simulink model "WaveletTraj"  (Simulink 10.1)
settings: Solver=FixedStepDiscrete  StartTime=0.0  StopTime=inf  FixedStep=Ts  RelTol=1e-3
PreLoadFcn:
  | load param
undefined symbols (not defined in the file or in its folder): c_maxsz, DiscIntNeverNeededParam, Dphival_fi, f, interp_gain, interp_uplim, phival_fi, Ts, tval_fi, w
libraries: simulink x36, dspsigops x24, dspindex x16, dspswit3 x12, simulink_extras x8
(part 3 of 4)

== system WaveletTraj/Wavelet Trajectory/TrajGen1/Compute Join Output/CalcRho ==
  tau : Inport
  tau1 : Inport  Port=2
  Constant : Constant  OutDataTypeStr=fixdt(1,w,f)
  Divide : Product  Inputs=*/  OutDataTypeStr=fixdt(1,w,f)  RndMeth=Nearest  SaturateOnIntegerOverflow=on
  Product : Product  OutDataTypeStr=fixdt(1,w,f)  RndMeth=Nearest  SaturateOnIntegerOverflow=on
  Saturation1 : Saturate  UpperLimit=2^(w-f-1)  LowerLimit=2^-f  OutDataTypeStr=fixdt(1,w,f)  RndMeth=Nearest
  Sum1 : Sum  Inputs=|+-  OutDataTypeStr=fixdt(1,w,f)  RndMeth=Nearest  SaturateOnIntegerOverflow=on
  Sum2 : Sum  Inputs=-+|  OutDataTypeStr=fixdt(1,w,f)  RndMeth=Nearest  SaturateOnIntegerOverflow=on
  Rho1 : Outport
  Rho2 : Outport  Port=2
  wires:
  Sum2/1 -> Rho2/1
  Saturation1/1 -> Divide/2
  Product/1 -> Sum2/1, Rho1/1
  Sum1/1 -> Product/2, Product/1
  Constant/1 -> Sum2/2, Sum1/2
  Divide/1 -> Sum1/1
  tau1/1 -> Saturation1/1
  tau/1 -> Divide/1

== system WaveletTraj/Wavelet Trajectory/TrajGen1/Compute Outputs/Compute Integral ==
  x : Inport
  max : Inport  Port=2
  min : Inport  Port=3
  Enable : EnablePort
  Compare To Zero : simulink/Logic and Bit Operations/Compare To Zero  SystemSampleTime=-1  relop=<  LogicOutDataTypeMode=boolean  ZeroCross=off
  Compare To Zero1 : simulink/Logic and Bit Operations/Compare To Zero  SystemSampleTime=-1  relop=>  LogicOutDataTypeMode=boolean  ZeroCross=off
  Discrete-Time Integrator : DiscreteIntegrator  IntegratorMethod=Integration: Trapezoidal  ExternalReset=level  InitialConditionSource=external  SampleTime=Ts  OutDataTypeStr=fixdt(1,w,f)  RndMeth=Nearest  SaturateOnIntegerOverflow=on  ICPrevOutput=DiscIntNeverNeededParam  ICPrevScaledInput=DiscIntNeverNeededParam
  Logical Operator : Logic  Operator=OR  IconShape=distinctive  AllPortsSameDT=off  OutDataTypeStr=boolean
  Logical Operator1 : Logic  IconShape=distinctive  AllPortsSameDT=off  OutDataTypeStr=boolean
  Logical Operator2 : Logic  IconShape=distinctive  AllPortsSameDT=off  OutDataTypeStr=boolean
  Logical Operator3 : Logic  Operator=OR  IconShape=distinctive  AllPortsSameDT=off  OutDataTypeStr=boolean
  Relational Operator1 : RelationalOperator  Operator=<=  OutDataTypeStr=boolean  RndMeth=Nearest
  Relational Operator2 : RelationalOperator  Operator=<=  OutDataTypeStr=boolean  RndMeth=Nearest
  S-R Flip-Flop : simulink_extras/Flip Flops/S-R Flip-Flop  SystemSampleTime=-1  initial_condition=0
  Sample and Hold1 : dspsigops/Sample and Hold  SystemSampleTime=-1  trig=Either edge  initCond=0  latchinput=off
  Sample and Hold2 : dspsigops/Sample and Hold  SystemSampleTime=-1  trig=Either edge  initCond=0  latchinput=off
  Saturation Dynamic : simulink/Discontinuities/Saturation Dynamic  SystemSampleTime=-1  OutMin=[]  OutMax=[]  OutDataTypeStr=fixdt(1,w,f)  OutputDataTypeScalingMode=Specify via dialog  OutDataType=fixdt(1,w,f)  OutScaling=[]  RndMeth=Nearest  DoSatur=on
  Terminator : Terminator
  Unit Delay : UnitDelay  SampleTime=-1
  Ix : Outport
  wires:
  max/1 -> Relational Operator1/1, Saturation Dynamic/1
  min/1 -> Relational Operator2/2, Saturation Dynamic/3
  Relational Operator1/1 -> Logical Operator/1, Sample and Hold1/1
  Relational Operator2/1 -> Sample and Hold2/1, Logical Operator/2
  Discrete-Time Integrator/1 -> Saturation Dynamic/2
  Saturation Dynamic/1 -> Ix/1, Unit Delay/1
  x/1 -> Discrete-Time Integrator/1, Compare To Zero/1, Compare To Zero1/1
  Unit Delay/1 -> Discrete-Time Integrator/3, Relational Operator1/2, Relational Operator2/1
  S-R Flip-Flop/1 -> Discrete-Time Integrator/2
  S-R Flip-Flop/2 -> Terminator/1
  Logical Operator/1 -> S-R Flip-Flop/1, Sample and Hold1/Trigger, Sample and Hold2/Trigger
  Compare To Zero/1 -> Logical Operator1/2
  Compare To Zero1/1 -> Logical Operator2/2
  Logical Operator1/1 -> Logical Operator3/1
  Logical Operator2/1 -> Logical Operator3/2
  Logical Operator3/1 -> S-R Flip-Flop/2
  Sample and Hold1/1 -> Logical Operator1/1
  Sample and Hold2/1 -> Logical Operator2/1

== system WaveletTraj/Wavelet Trajectory/TrajGen1/Compute Outputs/Rate Limiter1 ==
  up : Inport
  u : Inport  Port=2
  lo : Inport  Port=3
  Gain : Gain  Gain=1/Ts  ParamDataTypeStr=fixdt(1,w,f)  RndMeth=Nearest  SaturateOnIntegerOverflow=on  OutDataTypeStr=Inherit: Same as input
  Gain1 : Gain  Gain=Ts  ParamDataTypeStr=fixdt(1,w,f)  OutDataTypeStr=fixdt(1,w,f)  RndMeth=Nearest  SaturateOnIntegerOverflow=on
  Gain2 : Gain  Gain=Ts  ParamDataTypeStr=fixdt(1,w,f)  OutDataTypeStr=fixdt(1,w,f)  RndMeth=Nearest  SaturateOnIntegerOverflow=on
  Relational Operator : RelationalOperator  Operator=<  OutDataTypeStr=boolean  RndMeth=Nearest
  Relational Operator1 : RelationalOperator  Operator=>  OutDataTypeStr=boolean  RndMeth=Nearest
  Sum1 : Sum  Inputs=|++  OutDataTypeStr=fixdt(1,w,f)  RndMeth=Nearest  SaturateOnIntegerOverflow=on
  Sum2 : Sum  Inputs=|+-  OutDataTypeStr=fixdt(1,w,f)  RndMeth=Nearest  SaturateOnIntegerOverflow=on
  Sum3 : Sum  Inputs=|++  OutDataTypeStr=fixdt(1,w,f)  RndMeth=Nearest  SaturateOnIntegerOverflow=on
  Switch1 : Switch  Threshold=0.5  OutDataTypeStr=fixdt(1,w,f)  RndMeth=Nearest  SaturateOnIntegerOverflow=on
  Switch2 : Switch  Threshold=0.5  OutDataTypeStr=fixdt(1,w,f)  RndMeth=Nearest  SaturateOnIntegerOverflow=on
  Unit Delay : UnitDelay  SampleTime=-1
  y : Outport
  wires:
  u/1 -> Sum2/1, Switch1/3
  Sum2/1 -> Gain/1
  Unit Delay/1 -> Sum2/2, Sum1/2, Sum3/2
  Gain/1 -> Relational Operator/2, Relational Operator1/1
  up/1 -> Relational Operator/1, Gain1/1
  Relational Operator/1 -> Switch1/2
  Gain1/1 -> Sum1/1
  Sum1/1 -> Switch1/1
  Switch1/1 -> Switch2/1
  Switch2/1 -> y/1, Unit Delay/1
  Relational Operator1/1 -> Switch2/2
  lo/1 -> Relational Operator1/2, Gain2/1
  Gain2/1 -> Sum3/1
  Sum3/1 -> Switch2/3

== system WaveletTraj/Wavelet Trajectory/TrajGen1/Compute Outputs/Rate Limiter2 ==
  up : Inport
  u : Inport  Port=2
  lo : Inport  Port=3
  Gain : Gain  Gain=1/Ts  ParamDataTypeStr=fixdt(1,w,f)  RndMeth=Nearest  SaturateOnIntegerOverflow=on  OutDataTypeStr=Inherit: Same as input
  Gain1 : Gain  Gain=Ts  ParamDataTypeStr=fixdt(1,w,f)  OutDataTypeStr=fixdt(1,w,f)  RndMeth=Nearest  SaturateOnIntegerOverflow=on
  Gain2 : Gain  Gain=Ts  ParamDataTypeStr=fixdt(1,w,f)  OutDataTypeStr=fixdt(1,w,f)  RndMeth=Nearest  SaturateOnIntegerOverflow=on
  Relational Operator : RelationalOperator  Operator=<  OutDataTypeStr=boolean  RndMeth=Nearest
  Relational Operator1 : RelationalOperator  Operator=>  OutDataTypeStr=boolean  RndMeth=Nearest
  Sum1 : Sum  Inputs=|++  OutDataTypeStr=fixdt(1,w,f)  RndMeth=Nearest  SaturateOnIntegerOverflow=on
  Sum2 : Sum  Inputs=|+-  OutDataTypeStr=fixdt(1,w,f)  RndMeth=Nearest  SaturateOnIntegerOverflow=on
  Sum3 : Sum  Inputs=|++  OutDataTypeStr=fixdt(1,w,f)  RndMeth=Nearest  SaturateOnIntegerOverflow=on
  Switch1 : Switch  Threshold=0.5  OutDataTypeStr=fixdt(1,w,f)  RndMeth=Nearest  SaturateOnIntegerOverflow=on
  Switch2 : Switch  Threshold=0.5  OutDataTypeStr=fixdt(1,w,f)  RndMeth=Nearest  SaturateOnIntegerOverflow=on
  Unit Delay : UnitDelay  SampleTime=-1
  y : Outport
  wires:
  Sum3/1 -> Switch2/3
  Gain2/1 -> Sum3/1
  lo/1 -> Gain2/1, Relational Operator1/2
  Relational Operator1/1 -> Switch2/2
  Switch2/1 -> Unit Delay/1, y/1
  Switch1/1 -> Switch2/1
  Sum1/1 -> Switch1/1
  Gain1/1 -> Sum1/1
  Relational Operator/1 -> Switch1/2
  up/1 -> Gain1/1, Relational Operator/1
  Gain/1 -> Relational Operator1/1, Relational Operator/2
  Unit Delay/1 -> Sum3/2, Sum1/2, Sum2/2
  Sum2/1 -> Gain/1
  u/1 -> Switch1/3, Sum2/1

== system WaveletTraj/Wavelet Trajectory/TrajGen1/Compute Position/Position ==
  Res : Inport
  tau : Inport  Port=2
  c : Inport  Port=3
  N : Inport  Port=4
  Position : Subsystem  RTWFcnName=Trajectory_Position
  out : Outport
  wires:
  N/1 -> Position/4(N)
  c/1 -> Position/3(c)
  Position/1(out) -> out/1
  tau/1 -> Position/2(tau)
  Res/1 -> Position/1(Res)

== system WaveletTraj/Wavelet Trajectory/TrajGen1/Input Latching/Sample and Hold ==
  mode : Inport
  In : Inport  Port=2
  Trigger : TriggerPort  VariantControl=(inherit)  ZeroCross=off
  Constant : Constant  Value=2^3  OutDataTypeStr=fixdt(0,w,f)
  Constant1 : Constant  Value=2^4  OutDataTypeStr=fixdt(0,w,f)
  Data Type Conversion : DataTypeConversion  OutDataTypeStr=uint16  RndMeth=Ceiling  SaturateOnIntegerOverflow=on
  Multiport Switch : MultiPortSwitch  DataPortOrder=Zero-based contiguous  zeroidx=on  OutDataTypeStr=fixdt(0,w,f)  RndMeth=Nearest  SaturateOnIntegerOverflow=on
  " " : Outport  InitialOutput=initCond
  " 1" : Outport  Port=2  InitialOutput=initCond
  wires:
  Data Type Conversion/1 -> " 1"/1
  Multiport Switch/1 -> " "/1, Data Type Conversion/1
  mode/1 -> Multiport Switch/1
  In/1 -> Multiport Switch/2
  Constant/1 -> Multiport Switch/3
  Constant1/1 -> Multiport Switch/4

== system WaveletTraj/Wavelet Trajectory/TrajGen1/Input Latching/Sample and Hold2 ==
  In : Inport
  Trigger : TriggerPort  VariantControl=(inherit)  ZeroCross=off
  Data Type Conversion : DataTypeConversion  OutDataTypeStr=uint32  SaturateOnIntegerOverflow=on
  Gain : Gain  Gain=1/Ts  ParamDataTypeStr=fixdt(1,w,f)  OutDataTypeStr=fixdt(1,w,f)  RndMeth=Nearest  SaturateOnIntegerOverflow=on
  " " : Outport  InitialOutput=initCond
  wires:
  Data Type Conversion/1 -> " "/1
  Gain/1 -> Data Type Conversion/1
  In/1 -> Gain/1

== system WaveletTraj/Wavelet Trajectory/TrajGen1/Input Latching/Sample and Hold4 ==
  mode : Inport
  In : Inport  Port=2
  Trigger : TriggerPort  VariantControl=(inherit)  ZeroCross=off
  Multiport Switch : MultiPortSwitch  DataPortOrder=Zero-based contiguous  zeroidx=on  OutDataTypeStr=fixdt(1,w,f)  RndMeth=Nearest  SaturateOnIntegerOverflow=on
  constant : Constant  Value="[0.0156906989743308,  0.104549075132343,  0.277142440037961,  0.502199121925297,  0.726584938978675,  0.897421193763573,  0.982811374526835,  0.999579465917557,  1.00001660256494,  zeros(1,c_maxsz-9)]"  OutDataTypeStr=fixdt(1,w,f)
  constant1 : Constant  Value="[0.704980465851185,  0.994792363880808,  1.00001660256494*ones(1,15),  zeros(1,c_maxsz-17)]"  OutDataTypeStr=fixdt(1,w,f)
  " " : Outport  InitialOutput=initCond
  wires:
  Multiport Switch/1 -> " "/1
  mode/1 -> Multiport Switch/1
  In/1 -> Multiport Switch/2
  constant/1 -> Multiport Switch/3
  constant1/1 -> Multiport Switch/4

== system WaveletTraj/Wavelet Trajectory/TrajGen1/Input Latching/Sample and Hold5 ==
  mode : Inport
  x0 : Inport  Port=2
  xf : Inport  Port=3
  Trigger : TriggerPort  VariantControl=(inherit)  ZeroCross=off
  Constant : Constant  OutDataTypeStr=fixdt(1,w,f)
  Sum2 : Sum  Inputs=-+|  OutDataTypeStr=fixdt(1,w,f)  RndMeth=Nearest  SaturateOnIntegerOverflow=on
  Switch1 : Switch  Threshold=0.5  OutDataTypeStr=fixdt(1,w,f)  RndMeth=Nearest  SaturateOnIntegerOverflow=on
  " " : Outport  InitialOutput=initCond
  wires:
  x0/1 -> Sum2/1
  xf/1 -> Sum2/2
  mode/1 -> Switch1/2
  Sum2/1 -> Switch1/1
  Switch1/1 -> " "/1
  Constant/1 -> Switch1/3

== system WaveletTraj/Wavelet Trajectory/TrajGen2/Compute Join Coeffs/Derivative1 in tau ==
  Res : Inport
  tau : Inport  Port=2
  c : Inport  Port=3
  N : Inport  Port=4
  Derivative : Subsystem  RTWFcnName=Trajectory_Derivative
  out : Outport
  wires:
  Res/1 -> Derivative/1(Res)
  tau/1 -> Derivative/2(tau)
  Derivative/1(Dout) -> out/1
  c/1 -> Derivative/3(c)
  N/1 -> Derivative/4(N)

== system WaveletTraj/Wavelet Trajectory/TrajGen2/Compute Join Coeffs/Derivative2 in 0 ==
  Res : Inport
  tau : Inport  Port=2
  c : Inport  Port=3
  N : Inport  Port=4
  Derivative : Subsystem  RTWFcnName=Trajectory_Derivative
  out : Outport
  wires:
  N/1 -> Derivative/4(N)
  c/1 -> Derivative/3(c)
  Derivative/1(Dout) -> out/1
  tau/1 -> Derivative/2(tau)
  Res/1 -> Derivative/1(Res)

== system WaveletTraj/Wavelet Trajectory/TrajGen2/Compute Join Coeffs/Derivative2 in tau1 ==
  Res : Inport
  tau : Inport  Port=2
  c : Inport  Port=3
  N : Inport  Port=4
  Derivative : Subsystem  RTWFcnName=Trajectory_Derivative
  out : Outport
  wires:
  Res/1 -> Derivative/1(Res)
  tau/1 -> Derivative/2(tau)
  Derivative/1(Dout) -> out/1
  c/1 -> Derivative/3(c)
  N/1 -> Derivative/4(N)

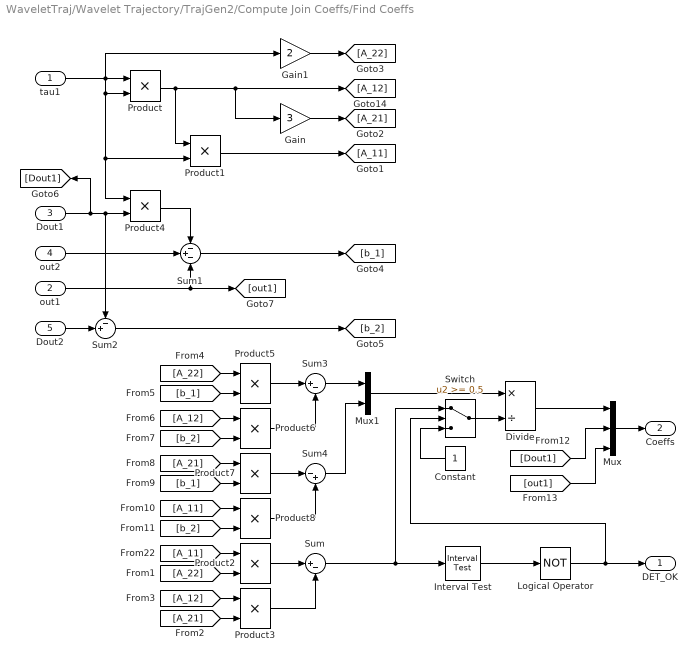
== system WaveletTraj/Wavelet Trajectory/TrajGen2/Compute Join Coeffs/Find Coeffs ==
  tau1 : Inport
  out1 : Inport  Port=2
  Dout1 : Inport  Port=3
  out2 : Inport  Port=4
  Dout2 : Inport  Port=5
  Constant : Constant  OutDataTypeStr=fixdt(1,w,f)
  Divide : Product  Inputs=*/  OutDataTypeStr=fixdt(1,w,f)  RndMeth=Nearest  SaturateOnIntegerOverflow=on
  Gain : Gain  Gain=3  RndMeth=Nearest  SaturateOnIntegerOverflow=on  OutDataTypeStr=Inherit: Same as input  ParamDataTypeStr=Inherit: Same as input
  Gain1 : Gain  Gain=2  RndMeth=Nearest  SaturateOnIntegerOverflow=on  OutDataTypeStr=Inherit: Same as input  ParamDataTypeStr=Inherit: Same as input
  Interval Test : simulink/Logic and Bit Operations/Interval Test  SystemSampleTime=-1  IntervalClosedRight=on  uplimit=2^-f  IntervalClosedLeft=on  lowlimit=-2^-f  LogicOutDataTypeMode=boolean
  Logical Operator : Logic  Operator=NOT  IconShape=distinctive  AllPortsSameDT=off  OutDataTypeStr=boolean
  Mux : Mux  Inputs=3
  Mux1 : Mux  Inputs=2
  Product{,1..8} (9 alike) : Product  OutDataTypeStr=fixdt(1,w,f)  RndMeth=Nearest  SaturateOnIntegerOverflow=on
  Sum : Sum  Inputs=|+-  OutDataTypeStr=fixdt(1,w,f)  RndMeth=Nearest  SaturateOnIntegerOverflow=on
  Sum1 : Sum  Inputs=-+-  OutDataTypeStr=fixdt(1,w,f)  RndMeth=Nearest  SaturateOnIntegerOverflow=on
  Sum2 : Sum  Inputs=-+|  OutDataTypeStr=fixdt(1,w,f)  RndMeth=Nearest  SaturateOnIntegerOverflow=on
  Sum3 : Sum  Inputs=|+-  OutDataTypeStr=fixdt(1,w,f)  RndMeth=Nearest  SaturateOnIntegerOverflow=on
  Sum4 : Sum  Inputs=|-+  OutDataTypeStr=fixdt(1,w,f)  RndMeth=Nearest  SaturateOnIntegerOverflow=on
  Switch : Switch  Threshold=0.5  OutDataTypeStr=fixdt(1,w,f)  RndMeth=Nearest  SaturateOnIntegerOverflow=on
  DET_OK : Outport
  Coeffs : Outport  Port=2
  wires:
  tau1/1 -> Product/1, Product/2, Product1/2, Product4/1, Gain1/1
  Product/1 -> Product1/1, [A_12], Gain/1
  Product1/1 -> [A_11]
  Gain/1 -> [A_21]
  Gain1/1 -> [A_22]
  [A_11] -> Product2/1
  [A_22] -> Product2/2
  [A_12] -> Product3/1
  [A_21] -> Product3/2
  Product2/1 -> Sum/1
  Product3/1 -> Sum/2
  Dout1/1 -> Product4/2, Sum2/1, [Dout1]
  out2/1 -> Sum1/2
  out1/1 -> Sum1/3, [out1]
  Product4/1 -> Sum1/1
  Dout2/1 -> Sum2/2
  Sum1/1 -> [b_1]
  Sum2/1 -> [b_2]
  [A_22] -> Product5/1
  [b_1] -> Product5/2
  [A_12] -> Product6/1
  [b_2] -> Product6/2
  Product5/1 -> Sum3/1
  Product6/1 -> Sum3/2
  [A_21] -> Product7/1
  [b_1] -> Product7/2
  [A_11] -> Product8/1
  [b_2] -> Product8/2
  Product7/1 -> Sum4/1
  Product8/1 -> Sum4/2
  Sum3/1 -> Mux1/1
  Sum4/1 -> Mux1/2
  Mux1/1 -> Divide/1
  Sum/1 -> Interval Test/1, Switch/1
  Divide/1 -> Mux/1
  [Dout1] -> Mux/2
  [out1] -> Mux/3
  Mux/1 -> Coeffs/1
  Interval Test/1 -> Logical Operator/1
  Logical Operator/1 -> DET_OK/1, Switch/2
  Switch/1 -> Divide/2
  Constant/1 -> Switch/3

== system WaveletTraj/Wavelet Trajectory/TrajGen2/Compute Join Coeffs/Position2 in tau1 ==
  Res : Inport
  tau : Inport  Port=2
  c : Inport  Port=3
  N : Inport  Port=4
  Position : Subsystem  RTWFcnName=Trajectory_Position
  out : Outport
  wires:
  N/1 -> Position/4(N)
  c/1 -> Position/3(c)
  Position/1(out) -> out/1
  tau/1 -> Position/2(tau)
  Res/1 -> Position/1(Res)

== system WaveletTraj/Wavelet Trajectory/TrajGen2/Compute Join Output/CalcPoly ==
  tau : Inport
  Coeffs : Inport  Port=2
  Add : Sum  Inputs=4  OutDataTypeStr=fixdt(1,w,f)  RndMeth=Nearest  SaturateOnIntegerOverflow=on
  Demux : Demux
  Product{,1..4} (5 alike) : Product  OutDataTypeStr=fixdt(1,w,f)  RndMeth=Nearest  SaturateOnIntegerOverflow=on
  out_poly3 : Outport
  wires:
  tau/1 -> Product/1, Product/2, Product1/2, Product4/1
  Product/1 -> Product1/1, Product3/1
  Product1/1 -> Product2/1
  Demux/1 -> Product2/2
  Demux/2 -> Product3/2
  Demux/3 -> Product4/2
  Product3/1 -> Add/1
  Product2/1 -> Add/2
  Product4/1 -> Add/3
  Demux/4 -> Add/4
  Add/1 -> out_poly3/1
  Coeffs/1 -> Demux/1

== system WaveletTraj/Wavelet Trajectory/TrajGen2/Compute Join Output/CalcRho ==
  tau : Inport
  tau1 : Inport  Port=2
  Constant : Constant  OutDataTypeStr=fixdt(1,w,f)
  Divide : Product  Inputs=*/  OutDataTypeStr=fixdt(1,w,f)  RndMeth=Nearest  SaturateOnIntegerOverflow=on
  Product : Product  OutDataTypeStr=fixdt(1,w,f)  RndMeth=Nearest  SaturateOnIntegerOverflow=on
  Saturation1 : Saturate  UpperLimit=2^(w-f-1)  LowerLimit=2^-f  OutDataTypeStr=fixdt(1,w,f)  RndMeth=Nearest
  Sum1 : Sum  Inputs=|+-  OutDataTypeStr=fixdt(1,w,f)  RndMeth=Nearest  SaturateOnIntegerOverflow=on
  Sum2 : Sum  Inputs=-+|  OutDataTypeStr=fixdt(1,w,f)  RndMeth=Nearest  SaturateOnIntegerOverflow=on
  Rho1 : Outport
  Rho2 : Outport  Port=2
  wires:
  tau/1 -> Divide/1
  tau1/1 -> Saturation1/1
  Divide/1 -> Sum1/1
  Constant/1 -> Sum1/2, Sum2/2
  Sum1/1 -> Product/1, Product/2
  Product/1 -> Rho1/1, Sum2/1
  Saturation1/1 -> Divide/2
  Sum2/1 -> Rho2/1

== system WaveletTraj/Wavelet Trajectory/TrajGen2/Compute Outputs/Compute Integral ==
  x : Inport
  max : Inport  Port=2
  min : Inport  Port=3
  Enable : EnablePort
  Compare To Zero : simulink/Logic and Bit Operations/Compare To Zero  SystemSampleTime=-1  relop=<  LogicOutDataTypeMode=boolean  ZeroCross=off
  Compare To Zero1 : simulink/Logic and Bit Operations/Compare To Zero  SystemSampleTime=-1  relop=>  LogicOutDataTypeMode=boolean  ZeroCross=off
  Discrete-Time Integrator : DiscreteIntegrator  IntegratorMethod=Integration: Trapezoidal  ExternalReset=level  InitialConditionSource=external  SampleTime=Ts  OutDataTypeStr=fixdt(1,w,f)  RndMeth=Nearest  SaturateOnIntegerOverflow=on  ICPrevOutput=DiscIntNeverNeededParam  ICPrevScaledInput=DiscIntNeverNeededParam
  Logical Operator : Logic  Operator=OR  IconShape=distinctive  AllPortsSameDT=off  OutDataTypeStr=boolean
  Logical Operator1 : Logic  IconShape=distinctive  AllPortsSameDT=off  OutDataTypeStr=boolean
  Logical Operator2 : Logic  IconShape=distinctive  AllPortsSameDT=off  OutDataTypeStr=boolean
  Logical Operator3 : Logic  Operator=OR  IconShape=distinctive  AllPortsSameDT=off  OutDataTypeStr=boolean
  Relational Operator1 : RelationalOperator  Operator=<=  OutDataTypeStr=boolean  RndMeth=Nearest
  Relational Operator2 : RelationalOperator  Operator=<=  OutDataTypeStr=boolean  RndMeth=Nearest
  S-R Flip-Flop : simulink_extras/Flip Flops/S-R Flip-Flop  SystemSampleTime=-1  initial_condition=0
  Sample and Hold1 : dspsigops/Sample and Hold  SystemSampleTime=-1  trig=Either edge  initCond=0  latchinput=off
  Sample and Hold2 : dspsigops/Sample and Hold  SystemSampleTime=-1  trig=Either edge  initCond=0  latchinput=off
  Saturation Dynamic : simulink/Discontinuities/Saturation Dynamic  SystemSampleTime=-1  OutMin=[]  OutMax=[]  OutDataTypeStr=fixdt(1,w,f)  OutputDataTypeScalingMode=Specify via dialog  OutDataType=fixdt(1,w,f)  OutScaling=[]  RndMeth=Nearest  DoSatur=on
  Terminator : Terminator
  Unit Delay : UnitDelay  SampleTime=-1
  Ix : Outport
  wires:
  Sample and Hold2/1 -> Logical Operator2/1
  Sample and Hold1/1 -> Logical Operator1/1
  Logical Operator3/1 -> S-R Flip-Flop/2
  Logical Operator2/1 -> Logical Operator3/2
  Logical Operator1/1 -> Logical Operator3/1
  Compare To Zero1/1 -> Logical Operator2/2
  Compare To Zero/1 -> Logical Operator1/2
  Logical Operator/1 -> Sample and Hold2/Trigger, Sample and Hold1/Trigger, S-R Flip-Flop/1
  S-R Flip-Flop/2 -> Terminator/1
  S-R Flip-Flop/1 -> Discrete-Time Integrator/2
  Unit Delay/1 -> Relational Operator2/1, Relational Operator1/2, Discrete-Time Integrator/3
  x/1 -> Compare To Zero1/1, Compare To Zero/1, Discrete-Time Integrator/1
  Saturation Dynamic/1 -> Unit Delay/1, Ix/1
  Discrete-Time Integrator/1 -> Saturation Dynamic/2
  Relational Operator2/1 -> Logical Operator/2, Sample and Hold2/1
  Relational Operator1/1 -> Sample and Hold1/1, Logical Operator/1
  min/1 -> Saturation Dynamic/3, Relational Operator2/2
  max/1 -> Saturation Dynamic/1, Relational Operator1/1

== system WaveletTraj/Wavelet Trajectory/TrajGen2/Compute Outputs/Rate Limiter1 ==
  up : Inport
  u : Inport  Port=2
  lo : Inport  Port=3
  Gain : Gain  Gain=1/Ts  ParamDataTypeStr=fixdt(1,w,f)  RndMeth=Nearest  SaturateOnIntegerOverflow=on  OutDataTypeStr=Inherit: Same as input
  Gain1 : Gain  Gain=Ts  ParamDataTypeStr=fixdt(1,w,f)  OutDataTypeStr=fixdt(1,w,f)  RndMeth=Nearest  SaturateOnIntegerOverflow=on
  Gain2 : Gain  Gain=Ts  ParamDataTypeStr=fixdt(1,w,f)  OutDataTypeStr=fixdt(1,w,f)  RndMeth=Nearest  SaturateOnIntegerOverflow=on
  Relational Operator : RelationalOperator  Operator=<  OutDataTypeStr=boolean  RndMeth=Nearest
  Relational Operator1 : RelationalOperator  Operator=>  OutDataTypeStr=boolean  RndMeth=Nearest
  Sum1 : Sum  Inputs=|++  OutDataTypeStr=fixdt(1,w,f)  RndMeth=Nearest  SaturateOnIntegerOverflow=on
  Sum2 : Sum  Inputs=|+-  OutDataTypeStr=fixdt(1,w,f)  RndMeth=Nearest  SaturateOnIntegerOverflow=on
  Sum3 : Sum  Inputs=|++  OutDataTypeStr=fixdt(1,w,f)  RndMeth=Nearest  SaturateOnIntegerOverflow=on
  Switch1 : Switch  Threshold=0.5  OutDataTypeStr=fixdt(1,w,f)  RndMeth=Nearest  SaturateOnIntegerOverflow=on
  Switch2 : Switch  Threshold=0.5  OutDataTypeStr=fixdt(1,w,f)  RndMeth=Nearest  SaturateOnIntegerOverflow=on
  Unit Delay : UnitDelay  SampleTime=-1
  y : Outport
  wires:
  Sum3/1 -> Switch2/3
  Gain2/1 -> Sum3/1
  lo/1 -> Gain2/1, Relational Operator1/2
  Relational Operator1/1 -> Switch2/2
  Switch2/1 -> Unit Delay/1, y/1
  Switch1/1 -> Switch2/1
  Sum1/1 -> Switch1/1
  Gain1/1 -> Sum1/1
  Relational Operator/1 -> Switch1/2
  up/1 -> Gain1/1, Relational Operator/1
  Gain/1 -> Relational Operator1/1, Relational Operator/2
  Unit Delay/1 -> Sum3/2, Sum1/2, Sum2/2
  Sum2/1 -> Gain/1
  u/1 -> Switch1/3, Sum2/1

== system WaveletTraj/Wavelet Trajectory/TrajGen2/Compute Outputs/Rate Limiter2 ==
  up : Inport
  u : Inport  Port=2
  lo : Inport  Port=3
  Gain : Gain  Gain=1/Ts  ParamDataTypeStr=fixdt(1,w,f)  RndMeth=Nearest  SaturateOnIntegerOverflow=on  OutDataTypeStr=Inherit: Same as input
  Gain1 : Gain  Gain=Ts  ParamDataTypeStr=fixdt(1,w,f)  OutDataTypeStr=fixdt(1,w,f)  RndMeth=Nearest  SaturateOnIntegerOverflow=on
  Gain2 : Gain  Gain=Ts  ParamDataTypeStr=fixdt(1,w,f)  OutDataTypeStr=fixdt(1,w,f)  RndMeth=Nearest  SaturateOnIntegerOverflow=on
  Relational Operator : RelationalOperator  Operator=<  OutDataTypeStr=boolean  RndMeth=Nearest
  Relational Operator1 : RelationalOperator  Operator=>  OutDataTypeStr=boolean  RndMeth=Nearest
  Sum1 : Sum  Inputs=|++  OutDataTypeStr=fixdt(1,w,f)  RndMeth=Nearest  SaturateOnIntegerOverflow=on
  Sum2 : Sum  Inputs=|+-  OutDataTypeStr=fixdt(1,w,f)  RndMeth=Nearest  SaturateOnIntegerOverflow=on
  Sum3 : Sum  Inputs=|++  OutDataTypeStr=fixdt(1,w,f)  RndMeth=Nearest  SaturateOnIntegerOverflow=on
  Switch1 : Switch  Threshold=0.5  OutDataTypeStr=fixdt(1,w,f)  RndMeth=Nearest  SaturateOnIntegerOverflow=on
  Switch2 : Switch  Threshold=0.5  OutDataTypeStr=fixdt(1,w,f)  RndMeth=Nearest  SaturateOnIntegerOverflow=on
  Unit Delay : UnitDelay  SampleTime=-1
  y : Outport
  wires:
  u/1 -> Sum2/1, Switch1/3
  Sum2/1 -> Gain/1
  Unit Delay/1 -> Sum2/2, Sum1/2, Sum3/2
  Gain/1 -> Relational Operator/2, Relational Operator1/1
  up/1 -> Relational Operator/1, Gain1/1
  Relational Operator/1 -> Switch1/2
  Gain1/1 -> Sum1/1
  Sum1/1 -> Switch1/1
  Switch1/1 -> Switch2/1
  Switch2/1 -> y/1, Unit Delay/1
  Relational Operator1/1 -> Switch2/2
  lo/1 -> Relational Operator1/2, Gain2/1
  Gain2/1 -> Sum3/1
  Sum3/1 -> Switch2/3

== system WaveletTraj/Wavelet Trajectory/TrajGen2/Compute Position/Position ==
  Res : Inport
  tau : Inport  Port=2
  c : Inport  Port=3
  N : Inport  Port=4
  Position : Subsystem  RTWFcnName=Trajectory_Position
  out : Outport
  wires:
  Res/1 -> Position/1(Res)
  tau/1 -> Position/2(tau)
  Position/1(out) -> out/1
  c/1 -> Position/3(c)
  N/1 -> Position/4(N)

== system WaveletTraj/Wavelet Trajectory/TrajGen2/Input Latching/Sample and Hold ==
  mode : Inport
  In : Inport  Port=2
  Trigger : TriggerPort  VariantControl=(inherit)  ZeroCross=off
  Constant : Constant  Value=2^3  OutDataTypeStr=fixdt(0,w,f)
  Constant1 : Constant  Value=2^4  OutDataTypeStr=fixdt(0,w,f)
  Data Type Conversion : DataTypeConversion  OutDataTypeStr=uint16  RndMeth=Ceiling  SaturateOnIntegerOverflow=on
  Multiport Switch : MultiPortSwitch  DataPortOrder=Zero-based contiguous  zeroidx=on  OutDataTypeStr=fixdt(0,w,f)  RndMeth=Nearest  SaturateOnIntegerOverflow=on
  " " : Outport  InitialOutput=initCond
  " 1" : Outport  Port=2  InitialOutput=initCond
  wires:
  Constant1/1 -> Multiport Switch/4
  Constant/1 -> Multiport Switch/3
  In/1 -> Multiport Switch/2
  mode/1 -> Multiport Switch/1
  Multiport Switch/1 -> Data Type Conversion/1, " "/1
  Data Type Conversion/1 -> " 1"/1

== system WaveletTraj/Wavelet Trajectory/TrajGen2/Input Latching/Sample and Hold2 ==
  In : Inport
  Trigger : TriggerPort  VariantControl=(inherit)  ZeroCross=off
  Data Type Conversion : DataTypeConversion  OutDataTypeStr=uint32  SaturateOnIntegerOverflow=on
  Gain : Gain  Gain=1/Ts  ParamDataTypeStr=fixdt(1,w,f)  OutDataTypeStr=fixdt(1,w,f)  RndMeth=Nearest  SaturateOnIntegerOverflow=on
  " " : Outport  InitialOutput=initCond
  wires:
  In/1 -> Gain/1
  Gain/1 -> Data Type Conversion/1
  Data Type Conversion/1 -> " "/1

== system WaveletTraj/Wavelet Trajectory/TrajGen2/Input Latching/Sample and Hold4 ==
  mode : Inport
  In : Inport  Port=2
  Trigger : TriggerPort  VariantControl=(inherit)  ZeroCross=off
  Multiport Switch : MultiPortSwitch  DataPortOrder=Zero-based contiguous  zeroidx=on  OutDataTypeStr=fixdt(1,w,f)  RndMeth=Nearest  SaturateOnIntegerOverflow=on
  constant : Constant  Value="[0.0156906989743308,  0.104549075132343,  0.277142440037961,  0.502199121925297,  0.726584938978675,  0.897421193763573,  0.982811374526835,  0.999579465917557,  1.00001660256494,  zeros(1,c_maxsz-9)]"  OutDataTypeStr=fixdt(1,w,f)
  constant1 : Constant  Value="[0.704980465851185,  0.994792363880808,  1.00001660256494*ones(1,15),  zeros(1,c_maxsz-17)]"  OutDataTypeStr=fixdt(1,w,f)
  " " : Outport  InitialOutput=initCond
  wires:
  constant1/1 -> Multiport Switch/4
  constant/1 -> Multiport Switch/3
  In/1 -> Multiport Switch/2
  mode/1 -> Multiport Switch/1
  Multiport Switch/1 -> " "/1

== system WaveletTraj/Wavelet Trajectory/TrajGen2/Input Latching/Sample and Hold5 ==
  mode : Inport
  x0 : Inport  Port=2
  xf : Inport  Port=3
  Trigger : TriggerPort  VariantControl=(inherit)  ZeroCross=off
  Constant : Constant  OutDataTypeStr=fixdt(1,w,f)
  Sum2 : Sum  Inputs=-+|  OutDataTypeStr=fixdt(1,w,f)  RndMeth=Nearest  SaturateOnIntegerOverflow=on
  Switch1 : Switch  Threshold=0.5  OutDataTypeStr=fixdt(1,w,f)  RndMeth=Nearest  SaturateOnIntegerOverflow=on
  " " : Outport  InitialOutput=initCond
  wires:
  Constant/1 -> Switch1/3
  Switch1/1 -> " "/1
  Sum2/1 -> Switch1/1
  mode/1 -> Switch1/2
  xf/1 -> Sum2/2
  x0/1 -> Sum2/1

== system WaveletTraj/Wavelet Trajectory/TrajGen3/Compute Join Coeffs/Derivative1 in tau ==
  Res : Inport
  tau : Inport  Port=2
  c : Inport  Port=3
  N : Inport  Port=4
  Derivative : Subsystem  RTWFcnName=Trajectory_Derivative
  out : Outport
  wires:
  N/1 -> Derivative/4(N)
  c/1 -> Derivative/3(c)
  Derivative/1(Dout) -> out/1
  tau/1 -> Derivative/2(tau)
  Res/1 -> Derivative/1(Res)

== system WaveletTraj/Wavelet Trajectory/TrajGen3/Compute Join Coeffs/Derivative2 in 0 ==
  Res : Inport
  tau : Inport  Port=2
  c : Inport  Port=3
  N : Inport  Port=4
  Derivative : Subsystem  RTWFcnName=Trajectory_Derivative
  out : Outport
  wires:
  Res/1 -> Derivative/1(Res)
  tau/1 -> Derivative/2(tau)
  Derivative/1(Dout) -> out/1
  c/1 -> Derivative/3(c)
  N/1 -> Derivative/4(N)

== system WaveletTraj/Wavelet Trajectory/TrajGen3/Compute Join Coeffs/Derivative2 in tau1 ==
  Res : Inport
  tau : Inport  Port=2
  c : Inport  Port=3
  N : Inport  Port=4
  Derivative : Subsystem  RTWFcnName=Trajectory_Derivative
  out : Outport
  wires:
  N/1 -> Derivative/4(N)
  c/1 -> Derivative/3(c)
  Derivative/1(Dout) -> out/1
  tau/1 -> Derivative/2(tau)
  Res/1 -> Derivative/1(Res)

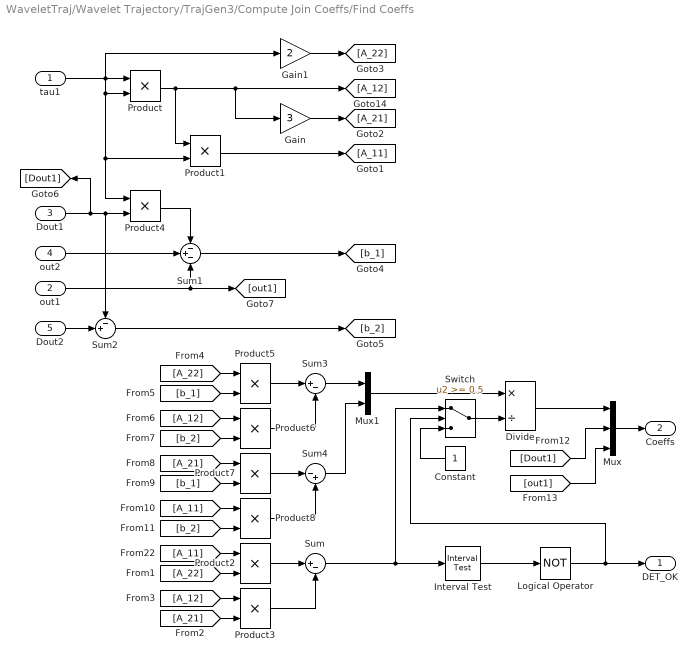
== system WaveletTraj/Wavelet Trajectory/TrajGen3/Compute Join Coeffs/Find Coeffs ==
  tau1 : Inport
  out1 : Inport  Port=2
  Dout1 : Inport  Port=3
  out2 : Inport  Port=4
  Dout2 : Inport  Port=5
  Constant : Constant  OutDataTypeStr=fixdt(1,w,f)
  Divide : Product  Inputs=*/  OutDataTypeStr=fixdt(1,w,f)  RndMeth=Nearest  SaturateOnIntegerOverflow=on
  Gain : Gain  Gain=3  RndMeth=Nearest  SaturateOnIntegerOverflow=on  OutDataTypeStr=Inherit: Same as input  ParamDataTypeStr=Inherit: Same as input
  Gain1 : Gain  Gain=2  RndMeth=Nearest  SaturateOnIntegerOverflow=on  OutDataTypeStr=Inherit: Same as input  ParamDataTypeStr=Inherit: Same as input
  Interval Test : simulink/Logic and Bit Operations/Interval Test  SystemSampleTime=-1  IntervalClosedRight=on  uplimit=2^-f  IntervalClosedLeft=on  lowlimit=-2^-f  LogicOutDataTypeMode=boolean
  Logical Operator : Logic  Operator=NOT  IconShape=distinctive  AllPortsSameDT=off  OutDataTypeStr=boolean
  Mux : Mux  Inputs=3
  Mux1 : Mux  Inputs=2
  Product{,1..8} (9 alike) : Product  OutDataTypeStr=fixdt(1,w,f)  RndMeth=Nearest  SaturateOnIntegerOverflow=on
  Sum : Sum  Inputs=|+-  OutDataTypeStr=fixdt(1,w,f)  RndMeth=Nearest  SaturateOnIntegerOverflow=on
  Sum1 : Sum  Inputs=-+-  OutDataTypeStr=fixdt(1,w,f)  RndMeth=Nearest  SaturateOnIntegerOverflow=on
  Sum2 : Sum  Inputs=-+|  OutDataTypeStr=fixdt(1,w,f)  RndMeth=Nearest  SaturateOnIntegerOverflow=on
  Sum3 : Sum  Inputs=|+-  OutDataTypeStr=fixdt(1,w,f)  RndMeth=Nearest  SaturateOnIntegerOverflow=on
  Sum4 : Sum  Inputs=|-+  OutDataTypeStr=fixdt(1,w,f)  RndMeth=Nearest  SaturateOnIntegerOverflow=on
  Switch : Switch  Threshold=0.5  OutDataTypeStr=fixdt(1,w,f)  RndMeth=Nearest  SaturateOnIntegerOverflow=on
  DET_OK : Outport
  Coeffs : Outport  Port=2
  wires:
  Constant/1 -> Switch/3
  Switch/1 -> Divide/2
  Logical Operator/1 -> Switch/2, DET_OK/1
  Interval Test/1 -> Logical Operator/1
  Mux/1 -> Coeffs/1
  [out1] -> Mux/3
  [Dout1] -> Mux/2
  Divide/1 -> Mux/1
  Sum/1 -> Switch/1, Interval Test/1
  Mux1/1 -> Divide/1
  Sum4/1 -> Mux1/2
  Sum3/1 -> Mux1/1
  Product8/1 -> Sum4/2
  Product7/1 -> Sum4/1
  [b_2] -> Product8/2
  [A_11] -> Product8/1
  [b_1] -> Product7/2
  [A_21] -> Product7/1
  Product6/1 -> Sum3/2
  Product5/1 -> Sum3/1
  [b_2] -> Product6/2
  [A_12] -> Product6/1
  [b_1] -> Product5/2
  [A_22] -> Product5/1
  Sum2/1 -> [b_2]
  Sum1/1 -> [b_1]
  Dout2/1 -> Sum2/2
  Product4/1 -> Sum1/1
  out1/1 -> [out1], Sum1/3
  out2/1 -> Sum1/2
  Dout1/1 -> [Dout1], Sum2/1, Product4/2
  Product3/1 -> Sum/2
  Product2/1 -> Sum/1
  [A_21] -> Product3/2
  [A_12] -> Product3/1
  [A_22] -> Product2/2
  [A_11] -> Product2/1
  Gain1/1 -> [A_22]
  Gain/1 -> [A_21]
  Product1/1 -> [A_11]
  Product/1 -> Gain/1, [A_12], Product1/1
  tau1/1 -> Gain1/1, Product4/1, Product1/2, Product/2, Product/1

== system WaveletTraj/Wavelet Trajectory/TrajGen3/Compute Join Coeffs/Position2 in tau1 ==
  Res : Inport
  tau : Inport  Port=2
  c : Inport  Port=3
  N : Inport  Port=4
  Position : Subsystem  RTWFcnName=Trajectory_Position
  out : Outport
  wires:
  Res/1 -> Position/1(Res)
  tau/1 -> Position/2(tau)
  Position/1(out) -> out/1
  c/1 -> Position/3(c)
  N/1 -> Position/4(N)

== system WaveletTraj/Wavelet Trajectory/TrajGen3/Compute Join Output/CalcPoly ==
  tau : Inport
  Coeffs : Inport  Port=2
  Add : Sum  Inputs=4  OutDataTypeStr=fixdt(1,w,f)  RndMeth=Nearest  SaturateOnIntegerOverflow=on
  Demux : Demux
  Product{,1..4} (5 alike) : Product  OutDataTypeStr=fixdt(1,w,f)  RndMeth=Nearest  SaturateOnIntegerOverflow=on
  out_poly3 : Outport
  wires:
  Coeffs/1 -> Demux/1
  Add/1 -> out_poly3/1
  Demux/4 -> Add/4
  Product4/1 -> Add/3
  Product2/1 -> Add/2
  Product3/1 -> Add/1
  Demux/3 -> Product4/2
  Demux/2 -> Product3/2
  Demux/1 -> Product2/2
  Product1/1 -> Product2/1
  Product/1 -> Product3/1, Product1/1
  tau/1 -> Product4/1, Product1/2, Product/2, Product/1

== system WaveletTraj/Wavelet Trajectory/TrajGen3/Compute Join Output/CalcRho ==
  tau : Inport
  tau1 : Inport  Port=2
  Constant : Constant  OutDataTypeStr=fixdt(1,w,f)
  Divide : Product  Inputs=*/  OutDataTypeStr=fixdt(1,w,f)  RndMeth=Nearest  SaturateOnIntegerOverflow=on
  Product : Product  OutDataTypeStr=fixdt(1,w,f)  RndMeth=Nearest  SaturateOnIntegerOverflow=on
  Saturation1 : Saturate  UpperLimit=2^(w-f-1)  LowerLimit=2^-f  OutDataTypeStr=fixdt(1,w,f)  RndMeth=Nearest
  Sum1 : Sum  Inputs=|+-  OutDataTypeStr=fixdt(1,w,f)  RndMeth=Nearest  SaturateOnIntegerOverflow=on
  Sum2 : Sum  Inputs=-+|  OutDataTypeStr=fixdt(1,w,f)  RndMeth=Nearest  SaturateOnIntegerOverflow=on
  Rho1 : Outport
  Rho2 : Outport  Port=2
  wires:
  Sum2/1 -> Rho2/1
  Saturation1/1 -> Divide/2
  Product/1 -> Sum2/1, Rho1/1
  Sum1/1 -> Product/2, Product/1
  Constant/1 -> Sum2/2, Sum1/2
  Divide/1 -> Sum1/1
  tau1/1 -> Saturation1/1
  tau/1 -> Divide/1

== system WaveletTraj/Wavelet Trajectory/TrajGen3/Compute Outputs/Compute Integral ==
  x : Inport
  max : Inport  Port=2
  min : Inport  Port=3
  Enable : EnablePort
  Compare To Zero : simulink/Logic and Bit Operations/Compare To Zero  SystemSampleTime=-1  relop=<  LogicOutDataTypeMode=boolean  ZeroCross=off
  Compare To Zero1 : simulink/Logic and Bit Operations/Compare To Zero  SystemSampleTime=-1  relop=>  LogicOutDataTypeMode=boolean  ZeroCross=off
  Discrete-Time Integrator : DiscreteIntegrator  IntegratorMethod=Integration: Trapezoidal  ExternalReset=level  InitialConditionSource=external  SampleTime=Ts  OutDataTypeStr=fixdt(1,w,f)  RndMeth=Nearest  SaturateOnIntegerOverflow=on  ICPrevOutput=DiscIntNeverNeededParam  ICPrevScaledInput=DiscIntNeverNeededParam
  Logical Operator : Logic  Operator=OR  IconShape=distinctive  AllPortsSameDT=off  OutDataTypeStr=boolean
  Logical Operator1 : Logic  IconShape=distinctive  AllPortsSameDT=off  OutDataTypeStr=boolean
  Logical Operator2 : Logic  IconShape=distinctive  AllPortsSameDT=off  OutDataTypeStr=boolean
  Logical Operator3 : Logic  Operator=OR  IconShape=distinctive  AllPortsSameDT=off  OutDataTypeStr=boolean
  Relational Operator1 : RelationalOperator  Operator=<=  OutDataTypeStr=boolean  RndMeth=Nearest
  Relational Operator2 : RelationalOperator  Operator=<=  OutDataTypeStr=boolean  RndMeth=Nearest
  S-R Flip-Flop : simulink_extras/Flip Flops/S-R Flip-Flop  SystemSampleTime=-1  initial_condition=0
  Sample and Hold1 : dspsigops/Sample and Hold  SystemSampleTime=-1  trig=Either edge  initCond=0  latchinput=off
  Sample and Hold2 : dspsigops/Sample and Hold  SystemSampleTime=-1  trig=Either edge  initCond=0  latchinput=off
  Saturation Dynamic : simulink/Discontinuities/Saturation Dynamic  SystemSampleTime=-1  OutMin=[]  OutMax=[]  OutDataTypeStr=fixdt(1,w,f)  OutputDataTypeScalingMode=Specify via dialog  OutDataType=fixdt(1,w,f)  OutScaling=[]  RndMeth=Nearest  DoSatur=on
  Terminator : Terminator
  Unit Delay : UnitDelay  SampleTime=-1
  Ix : Outport
  wires:
  max/1 -> Relational Operator1/1, Saturation Dynamic/1
  min/1 -> Relational Operator2/2, Saturation Dynamic/3
  Relational Operator1/1 -> Logical Operator/1, Sample and Hold1/1
  Relational Operator2/1 -> Sample and Hold2/1, Logical Operator/2
  Discrete-Time Integrator/1 -> Saturation Dynamic/2
  Saturation Dynamic/1 -> Ix/1, Unit Delay/1
  x/1 -> Discrete-Time Integrator/1, Compare To Zero/1, Compare To Zero1/1
  Unit Delay/1 -> Discrete-Time Integrator/3, Relational Operator1/2, Relational Operator2/1
  S-R Flip-Flop/1 -> Discrete-Time Integrator/2
  S-R Flip-Flop/2 -> Terminator/1
  Logical Operator/1 -> S-R Flip-Flop/1, Sample and Hold1/Trigger, Sample and Hold2/Trigger
  Compare To Zero/1 -> Logical Operator1/2
  Compare To Zero1/1 -> Logical Operator2/2
  Logical Operator1/1 -> Logical Operator3/1
  Logical Operator2/1 -> Logical Operator3/2
  Logical Operator3/1 -> S-R Flip-Flop/2
  Sample and Hold1/1 -> Logical Operator1/1
  Sample and Hold2/1 -> Logical Operator2/1

== system WaveletTraj/Wavelet Trajectory/TrajGen3/Compute Outputs/Rate Limiter1 ==
  up : Inport
  u : Inport  Port=2
  lo : Inport  Port=3
  Gain : Gain  Gain=1/Ts  ParamDataTypeStr=fixdt(1,w,f)  RndMeth=Nearest  SaturateOnIntegerOverflow=on  OutDataTypeStr=Inherit: Same as input
  Gain1 : Gain  Gain=Ts  ParamDataTypeStr=fixdt(1,w,f)  OutDataTypeStr=fixdt(1,w,f)  RndMeth=Nearest  SaturateOnIntegerOverflow=on
  Gain2 : Gain  Gain=Ts  ParamDataTypeStr=fixdt(1,w,f)  OutDataTypeStr=fixdt(1,w,f)  RndMeth=Nearest  SaturateOnIntegerOverflow=on
  Relational Operator : RelationalOperator  Operator=<  OutDataTypeStr=boolean  RndMeth=Nearest
  Relational Operator1 : RelationalOperator  Operator=>  OutDataTypeStr=boolean  RndMeth=Nearest
  Sum1 : Sum  Inputs=|++  OutDataTypeStr=fixdt(1,w,f)  RndMeth=Nearest  SaturateOnIntegerOverflow=on
  Sum2 : Sum  Inputs=|+-  OutDataTypeStr=fixdt(1,w,f)  RndMeth=Nearest  SaturateOnIntegerOverflow=on
  Sum3 : Sum  Inputs=|++  OutDataTypeStr=fixdt(1,w,f)  RndMeth=Nearest  SaturateOnIntegerOverflow=on
  Switch1 : Switch  Threshold=0.5  OutDataTypeStr=fixdt(1,w,f)  RndMeth=Nearest  SaturateOnIntegerOverflow=on
  Switch2 : Switch  Threshold=0.5  OutDataTypeStr=fixdt(1,w,f)  RndMeth=Nearest  SaturateOnIntegerOverflow=on
  Unit Delay : UnitDelay  SampleTime=-1
  y : Outport
  wires:
  u/1 -> Sum2/1, Switch1/3
  Sum2/1 -> Gain/1
  Unit Delay/1 -> Sum2/2, Sum1/2, Sum3/2
  Gain/1 -> Relational Operator/2, Relational Operator1/1
  up/1 -> Relational Operator/1, Gain1/1
  Relational Operator/1 -> Switch1/2
  Gain1/1 -> Sum1/1
  Sum1/1 -> Switch1/1
  Switch1/1 -> Switch2/1
  Switch2/1 -> y/1, Unit Delay/1
  Relational Operator1/1 -> Switch2/2
  lo/1 -> Relational Operator1/2, Gain2/1
  Gain2/1 -> Sum3/1
  Sum3/1 -> Switch2/3

== system WaveletTraj/Wavelet Trajectory/TrajGen3/Compute Outputs/Rate Limiter2 ==
  up : Inport
  u : Inport  Port=2
  lo : Inport  Port=3
  Gain : Gain  Gain=1/Ts  ParamDataTypeStr=fixdt(1,w,f)  RndMeth=Nearest  SaturateOnIntegerOverflow=on  OutDataTypeStr=Inherit: Same as input
  Gain1 : Gain  Gain=Ts  ParamDataTypeStr=fixdt(1,w,f)  OutDataTypeStr=fixdt(1,w,f)  RndMeth=Nearest  SaturateOnIntegerOverflow=on
  Gain2 : Gain  Gain=Ts  ParamDataTypeStr=fixdt(1,w,f)  OutDataTypeStr=fixdt(1,w,f)  RndMeth=Nearest  SaturateOnIntegerOverflow=on
  Relational Operator : RelationalOperator  Operator=<  OutDataTypeStr=boolean  RndMeth=Nearest
  Relational Operator1 : RelationalOperator  Operator=>  OutDataTypeStr=boolean  RndMeth=Nearest
  Sum1 : Sum  Inputs=|++  OutDataTypeStr=fixdt(1,w,f)  RndMeth=Nearest  SaturateOnIntegerOverflow=on
  Sum2 : Sum  Inputs=|+-  OutDataTypeStr=fixdt(1,w,f)  RndMeth=Nearest  SaturateOnIntegerOverflow=on
  Sum3 : Sum  Inputs=|++  OutDataTypeStr=fixdt(1,w,f)  RndMeth=Nearest  SaturateOnIntegerOverflow=on
  Switch1 : Switch  Threshold=0.5  OutDataTypeStr=fixdt(1,w,f)  RndMeth=Nearest  SaturateOnIntegerOverflow=on
  Switch2 : Switch  Threshold=0.5  OutDataTypeStr=fixdt(1,w,f)  RndMeth=Nearest  SaturateOnIntegerOverflow=on
  Unit Delay : UnitDelay  SampleTime=-1
  y : Outport
  wires:
  Sum3/1 -> Switch2/3
  Gain2/1 -> Sum3/1
  lo/1 -> Gain2/1, Relational Operator1/2
  Relational Operator1/1 -> Switch2/2
  Switch2/1 -> Unit Delay/1, y/1
  Switch1/1 -> Switch2/1
  Sum1/1 -> Switch1/1
  Gain1/1 -> Sum1/1
  Relational Operator/1 -> Switch1/2
  up/1 -> Gain1/1, Relational Operator/1
  Gain/1 -> Relational Operator1/1, Relational Operator/2
  Unit Delay/1 -> Sum3/2, Sum1/2, Sum2/2
  Sum2/1 -> Gain/1
  u/1 -> Switch1/3, Sum2/1

== system WaveletTraj/Wavelet Trajectory/TrajGen3/Compute Position/Position ==
  Res : Inport
  tau : Inport  Port=2
  c : Inport  Port=3
  N : Inport  Port=4
  Position : Subsystem  RTWFcnName=Trajectory_Position
  out : Outport
  wires:
  N/1 -> Position/4(N)
  c/1 -> Position/3(c)
  Position/1(out) -> out/1
  tau/1 -> Position/2(tau)
  Res/1 -> Position/1(Res)

== system WaveletTraj/Wavelet Trajectory/TrajGen3/Input Latching/Sample and Hold ==
  mode : Inport
  In : Inport  Port=2
  Trigger : TriggerPort  VariantControl=(inherit)  ZeroCross=off
  Constant : Constant  Value=2^3  OutDataTypeStr=fixdt(0,w,f)
  Constant1 : Constant  Value=2^4  OutDataTypeStr=fixdt(0,w,f)
  Data Type Conversion : DataTypeConversion  OutDataTypeStr=uint16  RndMeth=Ceiling  SaturateOnIntegerOverflow=on
  Multiport Switch : MultiPortSwitch  DataPortOrder=Zero-based contiguous  zeroidx=on  OutDataTypeStr=fixdt(0,w,f)  RndMeth=Nearest  SaturateOnIntegerOverflow=on
  " " : Outport  InitialOutput=initCond
  " 1" : Outport  Port=2  InitialOutput=initCond
  wires:
  Data Type Conversion/1 -> " 1"/1
  Multiport Switch/1 -> " "/1, Data Type Conversion/1
  mode/1 -> Multiport Switch/1
  In/1 -> Multiport Switch/2
  Constant/1 -> Multiport Switch/3
  Constant1/1 -> Multiport Switch/4

== system WaveletTraj/Wavelet Trajectory/TrajGen3/Input Latching/Sample and Hold2 ==
  In : Inport
  Trigger : TriggerPort  VariantControl=(inherit)  ZeroCross=off
  Data Type Conversion : DataTypeConversion  OutDataTypeStr=uint32  SaturateOnIntegerOverflow=on
  Gain : Gain  Gain=1/Ts  ParamDataTypeStr=fixdt(1,w,f)  OutDataTypeStr=fixdt(1,w,f)  RndMeth=Nearest  SaturateOnIntegerOverflow=on
  " " : Outport  InitialOutput=initCond
  wires:
  Data Type Conversion/1 -> " "/1
  Gain/1 -> Data Type Conversion/1
  In/1 -> Gain/1

== system WaveletTraj/Wavelet Trajectory/TrajGen3/Input Latching/Sample and Hold4 ==
  mode : Inport
  In : Inport  Port=2
  Trigger : TriggerPort  VariantControl=(inherit)  ZeroCross=off
  Multiport Switch : MultiPortSwitch  DataPortOrder=Zero-based contiguous  zeroidx=on  OutDataTypeStr=fixdt(1,w,f)  RndMeth=Nearest  SaturateOnIntegerOverflow=on
  constant : Constant  Value="[0.0156906989743308,  0.104549075132343,  0.277142440037961,  0.502199121925297,  0.726584938978675,  0.897421193763573,  0.982811374526835,  0.999579465917557,  1.00001660256494,  zeros(1,c_maxsz-9)]"  OutDataTypeStr=fixdt(1,w,f)
  constant1 : Constant  Value="[0.704980465851185,  0.994792363880808,  1.00001660256494*ones(1,15),  zeros(1,c_maxsz-17)]"  OutDataTypeStr=fixdt(1,w,f)
  " " : Outport  InitialOutput=initCond
  wires:
  Multiport Switch/1 -> " "/1
  mode/1 -> Multiport Switch/1
  In/1 -> Multiport Switch/2
  constant/1 -> Multiport Switch/3
  constant1/1 -> Multiport Switch/4

== system WaveletTraj/Wavelet Trajectory/TrajGen3/Input Latching/Sample and Hold5 ==
  mode : Inport
  x0 : Inport  Port=2
  xf : Inport  Port=3
  Trigger : TriggerPort  VariantControl=(inherit)  ZeroCross=off
  Constant : Constant  OutDataTypeStr=fixdt(1,w,f)
  Sum2 : Sum  Inputs=-+|  OutDataTypeStr=fixdt(1,w,f)  RndMeth=Nearest  SaturateOnIntegerOverflow=on
  Switch1 : Switch  Threshold=0.5  OutDataTypeStr=fixdt(1,w,f)  RndMeth=Nearest  SaturateOnIntegerOverflow=on
  " " : Outport  InitialOutput=initCond
  wires:
  x0/1 -> Sum2/1
  xf/1 -> Sum2/2
  mode/1 -> Switch1/2
  Sum2/1 -> Switch1/1
  Switch1/1 -> " "/1
  Constant/1 -> Switch1/3

== system WaveletTraj/Wavelet Trajectory/TrajGen4/Compute Join Coeffs/Derivative1 in tau ==
  Res : Inport
  tau : Inport  Port=2
  c : Inport  Port=3
  N : Inport  Port=4
  Derivative : Subsystem  RTWFcnName=Trajectory_Derivative
  out : Outport
  wires:
  Res/1 -> Derivative/1(Res)
  tau/1 -> Derivative/2(tau)
  Derivative/1(Dout) -> out/1
  c/1 -> Derivative/3(c)
  N/1 -> Derivative/4(N)

== system WaveletTraj/Wavelet Trajectory/TrajGen4/Compute Join Coeffs/Derivative2 in 0 ==
  Res : Inport
  tau : Inport  Port=2
  c : Inport  Port=3
  N : Inport  Port=4
  Derivative : Subsystem  RTWFcnName=Trajectory_Derivative
  out : Outport
  wires:
  N/1 -> Derivative/4(N)
  c/1 -> Derivative/3(c)
  Derivative/1(Dout) -> out/1
  tau/1 -> Derivative/2(tau)
  Res/1 -> Derivative/1(Res)

== system WaveletTraj/Wavelet Trajectory/TrajGen4/Compute Join Coeffs/Derivative2 in tau1 ==
  Res : Inport
  tau : Inport  Port=2
  c : Inport  Port=3
  N : Inport  Port=4
  Derivative : Subsystem  RTWFcnName=Trajectory_Derivative
  out : Outport
  wires:
  Res/1 -> Derivative/1(Res)
  tau/1 -> Derivative/2(tau)
  Derivative/1(Dout) -> out/1
  c/1 -> Derivative/3(c)
  N/1 -> Derivative/4(N)

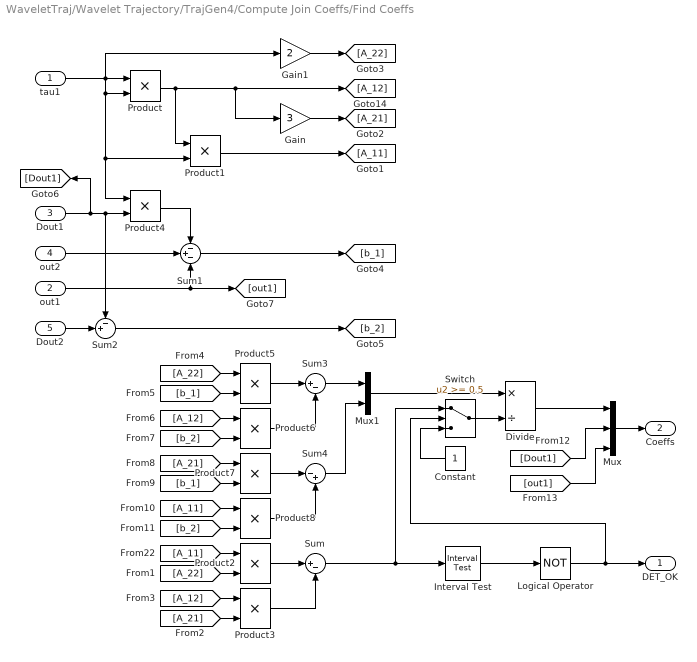
== system WaveletTraj/Wavelet Trajectory/TrajGen4/Compute Join Coeffs/Find Coeffs ==
  tau1 : Inport
  out1 : Inport  Port=2
  Dout1 : Inport  Port=3
  out2 : Inport  Port=4
  Dout2 : Inport  Port=5
  Constant : Constant  OutDataTypeStr=fixdt(1,w,f)
  Divide : Product  Inputs=*/  OutDataTypeStr=fixdt(1,w,f)  RndMeth=Nearest  SaturateOnIntegerOverflow=on
  Gain : Gain  Gain=3  RndMeth=Nearest  SaturateOnIntegerOverflow=on  OutDataTypeStr=Inherit: Same as input  ParamDataTypeStr=Inherit: Same as input
  Gain1 : Gain  Gain=2  RndMeth=Nearest  SaturateOnIntegerOverflow=on  OutDataTypeStr=Inherit: Same as input  ParamDataTypeStr=Inherit: Same as input
  Interval Test : simulink/Logic and Bit Operations/Interval Test  SystemSampleTime=-1  IntervalClosedRight=on  uplimit=2^-f  IntervalClosedLeft=on  lowlimit=-2^-f  LogicOutDataTypeMode=boolean
  Logical Operator : Logic  Operator=NOT  IconShape=distinctive  AllPortsSameDT=off  OutDataTypeStr=boolean
  Mux : Mux  Inputs=3
  Mux1 : Mux  Inputs=2
  Product{,1..8} (9 alike) : Product  OutDataTypeStr=fixdt(1,w,f)  RndMeth=Nearest  SaturateOnIntegerOverflow=on
  Sum : Sum  Inputs=|+-  OutDataTypeStr=fixdt(1,w,f)  RndMeth=Nearest  SaturateOnIntegerOverflow=on
  Sum1 : Sum  Inputs=-+-  OutDataTypeStr=fixdt(1,w,f)  RndMeth=Nearest  SaturateOnIntegerOverflow=on
  Sum2 : Sum  Inputs=-+|  OutDataTypeStr=fixdt(1,w,f)  RndMeth=Nearest  SaturateOnIntegerOverflow=on
  Sum3 : Sum  Inputs=|+-  OutDataTypeStr=fixdt(1,w,f)  RndMeth=Nearest  SaturateOnIntegerOverflow=on
  Sum4 : Sum  Inputs=|-+  OutDataTypeStr=fixdt(1,w,f)  RndMeth=Nearest  SaturateOnIntegerOverflow=on
  Switch : Switch  Threshold=0.5  OutDataTypeStr=fixdt(1,w,f)  RndMeth=Nearest  SaturateOnIntegerOverflow=on
  DET_OK : Outport
  Coeffs : Outport  Port=2
  wires:
  tau1/1 -> Product/1, Product/2, Product1/2, Product4/1, Gain1/1
  Product/1 -> Product1/1, [A_12], Gain/1
  Product1/1 -> [A_11]
  Gain/1 -> [A_21]
  Gain1/1 -> [A_22]
  [A_11] -> Product2/1
  [A_22] -> Product2/2
  [A_12] -> Product3/1
  [A_21] -> Product3/2
  Product2/1 -> Sum/1
  Product3/1 -> Sum/2
  Dout1/1 -> Product4/2, Sum2/1, [Dout1]
  out2/1 -> Sum1/2
  out1/1 -> Sum1/3, [out1]
  Product4/1 -> Sum1/1
  Dout2/1 -> Sum2/2
  Sum1/1 -> [b_1]
  Sum2/1 -> [b_2]
  [A_22] -> Product5/1
  [b_1] -> Product5/2
  [A_12] -> Product6/1
  [b_2] -> Product6/2
  Product5/1 -> Sum3/1
  Product6/1 -> Sum3/2
  [A_21] -> Product7/1
  [b_1] -> Product7/2
  [A_11] -> Product8/1
  [b_2] -> Product8/2
  Product7/1 -> Sum4/1
  Product8/1 -> Sum4/2
  Sum3/1 -> Mux1/1
  Sum4/1 -> Mux1/2
  Mux1/1 -> Divide/1
  Sum/1 -> Interval Test/1, Switch/1
  Divide/1 -> Mux/1
  [Dout1] -> Mux/2
  [out1] -> Mux/3
  Mux/1 -> Coeffs/1
  Interval Test/1 -> Logical Operator/1
  Logical Operator/1 -> DET_OK/1, Switch/2
  Switch/1 -> Divide/2
  Constant/1 -> Switch/3

== system WaveletTraj/Wavelet Trajectory/TrajGen4/Compute Join Coeffs/Position2 in tau1 ==
  Res : Inport
  tau : Inport  Port=2
  c : Inport  Port=3
  N : Inport  Port=4
  Position : Subsystem  RTWFcnName=Trajectory_Position
  out : Outport
  wires:
  N/1 -> Position/4(N)
  c/1 -> Position/3(c)
  Position/1(out) -> out/1
  tau/1 -> Position/2(tau)
  Res/1 -> Position/1(Res)

== system WaveletTraj/Wavelet Trajectory/TrajGen4/Compute Join Output/CalcPoly ==
  tau : Inport
  Coeffs : Inport  Port=2
  Add : Sum  Inputs=4  OutDataTypeStr=fixdt(1,w,f)  RndMeth=Nearest  SaturateOnIntegerOverflow=on
  Demux : Demux
  Product{,1..4} (5 alike) : Product  OutDataTypeStr=fixdt(1,w,f)  RndMeth=Nearest  SaturateOnIntegerOverflow=on
  out_poly3 : Outport
  wires:
  tau/1 -> Product/1, Product/2, Product1/2, Product4/1
  Product/1 -> Product1/1, Product3/1
  Product1/1 -> Product2/1
  Demux/1 -> Product2/2
  Demux/2 -> Product3/2
  Demux/3 -> Product4/2
  Product3/1 -> Add/1
  Product2/1 -> Add/2
  Product4/1 -> Add/3
  Demux/4 -> Add/4
  Add/1 -> out_poly3/1
  Coeffs/1 -> Demux/1

== system WaveletTraj/Wavelet Trajectory/TrajGen4/Compute Join Output/CalcRho ==
  tau : Inport
  tau1 : Inport  Port=2
  Constant : Constant  OutDataTypeStr=fixdt(1,w,f)
  Divide : Product  Inputs=*/  OutDataTypeStr=fixdt(1,w,f)  RndMeth=Nearest  SaturateOnIntegerOverflow=on
  Product : Product  OutDataTypeStr=fixdt(1,w,f)  RndMeth=Nearest  SaturateOnIntegerOverflow=on
  Saturation1 : Saturate  UpperLimit=2^(w-f-1)  LowerLimit=2^-f  OutDataTypeStr=fixdt(1,w,f)  RndMeth=Nearest
  Sum1 : Sum  Inputs=|+-  OutDataTypeStr=fixdt(1,w,f)  RndMeth=Nearest  SaturateOnIntegerOverflow=on
  Sum2 : Sum  Inputs=-+|  OutDataTypeStr=fixdt(1,w,f)  RndMeth=Nearest  SaturateOnIntegerOverflow=on
  Rho1 : Outport
  Rho2 : Outport  Port=2
  wires:
  tau/1 -> Divide/1
  tau1/1 -> Saturation1/1
  Divide/1 -> Sum1/1
  Constant/1 -> Sum1/2, Sum2/2
  Sum1/1 -> Product/1, Product/2
  Product/1 -> Rho1/1, Sum2/1
  Saturation1/1 -> Divide/2
  Sum2/1 -> Rho2/1
